simulink model "nouveaux_graphes2"  (R2018a)
settings: Solver=VariableStepAuto  StartTime=0.0  StopTime=100  RelTol=1e-3
settings Model: Creator=acer  LastModifiedBy=ITEC

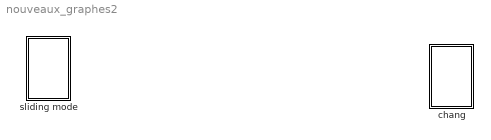
== system nouveaux_graphes2 ==
  chang : Subsystem
  sliding mode : Subsystem

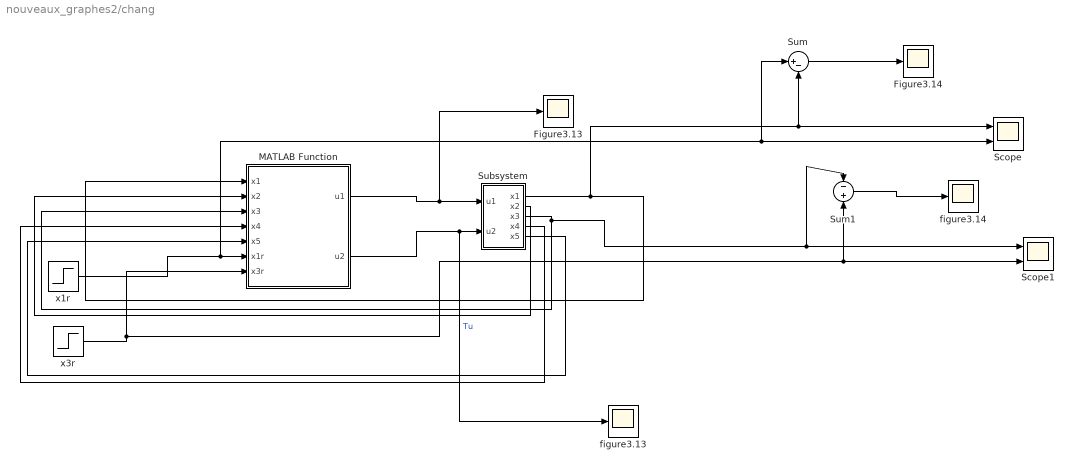
== system nouveaux_graphes2/chang ==
  Figure3.13 : Scope
  Figure3.14 : Scope
  MATLAB Function : MATLAB Function  TreatAsAtomicUnit=on
  Scope : Scope  NumInputPorts=2
  Scope1 : Scope  NumInputPorts=2
  Subsystem : Subsystem
  Sum : Sum  Inputs=|+-
  Sum1 : Sum  Inputs=-+
  figure3.13 : Scope
  figure3.14 : Scope
  x1r : Step  Time=0  After=8*10^6  SampleTime=0
  x3r : Step  Time=0  After=0.36  SampleTime=0
  wires:
  Subsystem/1(x1) -> Sum/2, Scope/1, MATLAB Function/1(x1)
  Subsystem/4(x4) -> MATLAB Function/4(x4)
  Subsystem/5(x5) -> MATLAB Function/5(x5)
  Subsystem/2(x2) -> MATLAB Function/2(x2)
  x1r/1 -> Sum/1, Scope/2, MATLAB Function/6(x1r)
  Sum/1 -> Figure3.14/1
  Subsystem/3(x3) -> Sum1/1, Scope1/1, MATLAB Function/3(x3)
  x3r/1 -> Sum1/2, Scope1/2, MATLAB Function/7(x3r)
  Sum1/1 -> figure3.14/1
  MATLAB Function/1(u1) -> Figure3.13/1, Subsystem/1(u1)
  MATLAB Function/2(u2) -> figure3.13/1, Subsystem/2(u2)  "Tu"

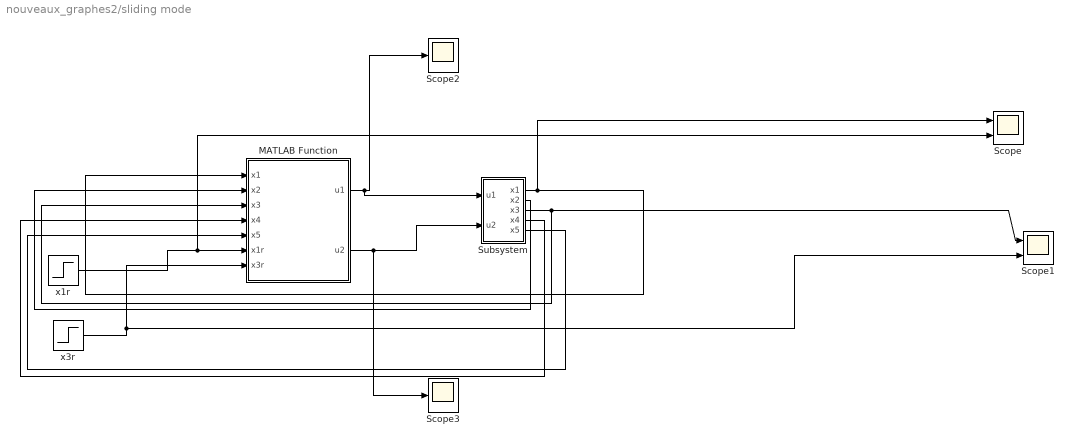
== system nouveaux_graphes2/sliding mode ==
  MATLAB Function : MATLAB Function  TreatAsAtomicUnit=on
  Scope : Scope  NumInputPorts=2
  Scope1 : Scope  NumInputPorts=2
  Scope2 : Scope
  Scope3 : Scope
  Subsystem : Subsystem
  x1r : Step  Time=0  After=8*10^6  SampleTime=0
  x3r : Step  Time=0  After=0.36  SampleTime=0
  wires:
  Subsystem/2(x2) -> MATLAB Function/2(x2)
  Subsystem/1(x1) -> MATLAB Function/1(x1), Scope/1
  MATLAB Function/2(u2) -> Scope3/1, Subsystem/2(u2)
  Subsystem/5(x5) -> MATLAB Function/5(x5)
  x3r/1 -> Scope1/2, MATLAB Function/7(x3r)
  Subsystem/3(x3) -> MATLAB Function/3(x3), Scope1/1
  Subsystem/4(x4) -> MATLAB Function/4(x4)
  x1r/1 -> Scope/2, MATLAB Function/6(x1r)
  MATLAB Function/1(u1) -> Subsystem/1(u1), Scope2/1

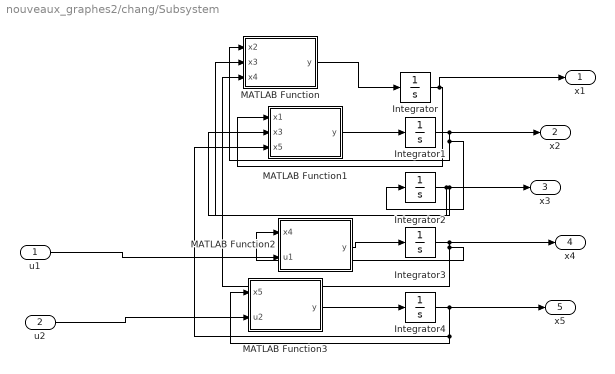
== system nouveaux_graphes2/chang/Subsystem ==
  u1 : Inport
  u2 : Inport  Port=2
  Integrator{,1..4} (5 alike) : Integrator
  MATLAB Function : MATLAB Function  TreatAsAtomicUnit=on
  MATLAB Function1 : MATLAB Function  TreatAsAtomicUnit=on
  MATLAB Function2 : MATLAB Function  TreatAsAtomicUnit=on
  MATLAB Function3 : MATLAB Function  TreatAsAtomicUnit=on
  x1 : Outport
  x2 : Outport  Port=2
  x3 : Outport  Port=3
  x4 : Outport  Port=4
  x5 : Outport  Port=5
  wires:
  Integrator/1 -> x1/1, MATLAB Function1/1(x1)
  Integrator1/1 -> x2/1, Integrator2/1, MATLAB Function/1(x2)
  MATLAB Function3/1(y) -> Integrator4/1
  MATLAB Function1/1(y) -> Integrator1/1
  u1/1 -> MATLAB Function2/2(u1)
  Integrator2/1 -> MATLAB Function1/2(x3), x3/1, MATLAB Function/2(x3)
  Integrator3/1 -> x4/1, MATLAB Function2/1(x4), MATLAB Function/3(x4)
  MATLAB Function2/1(y) -> Integrator3/1
  Integrator4/1 -> x5/1, MATLAB Function3/1(x5), MATLAB Function1/3(x5)
  MATLAB Function/1(y) -> Integrator/1
  u2/1 -> MATLAB Function3/2(u2)

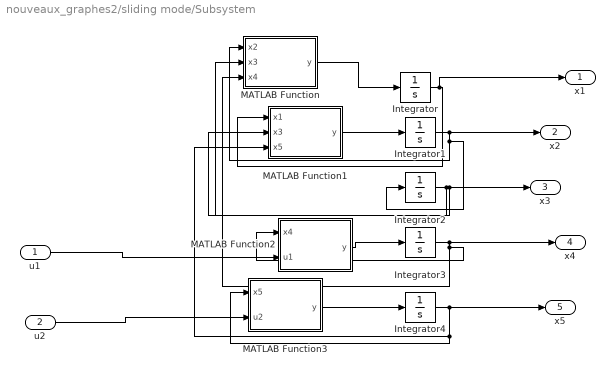
== system nouveaux_graphes2/sliding mode/Subsystem ==
  u1 : Inport
  u2 : Inport  Port=2
  Integrator{,1..4} (5 alike) : Integrator
  MATLAB Function : MATLAB Function  TreatAsAtomicUnit=on
  MATLAB Function1 : MATLAB Function  TreatAsAtomicUnit=on
  MATLAB Function2 : MATLAB Function  TreatAsAtomicUnit=on
  MATLAB Function3 : MATLAB Function  TreatAsAtomicUnit=on
  x1 : Outport
  x2 : Outport  Port=2
  x3 : Outport  Port=3
  x4 : Outport  Port=4
  x5 : Outport  Port=5
  wires:
  Integrator/1 -> x1/1, MATLAB Function1/1(x1)
  Integrator1/1 -> x2/1, Integrator2/1, MATLAB Function/1(x2)
  MATLAB Function3/1(y) -> Integrator4/1
  MATLAB Function1/1(y) -> Integrator1/1
  u1/1 -> MATLAB Function2/2(u1)
  Integrator2/1 -> MATLAB Function1/2(x3), x3/1, MATLAB Function/2(x3)
  Integrator3/1 -> x4/1, MATLAB Function2/1(x4), MATLAB Function/3(x4)
  MATLAB Function2/1(y) -> Integrator3/1
  Integrator4/1 -> x5/1, MATLAB Function3/1(x5), MATLAB Function1/3(x5)
  MATLAB Function/1(y) -> Integrator/1
  u2/1 -> MATLAB Function3/2(u2)

== matlab function nouveaux_graphes2/sliding mode/Subsystem/MATLAB Function1 ==
  data: x1 input; y output; x3 input; x5 input
function y = fcn(x1,x3,x5)
g = 9.8;
rau = 7800;
L = 5.8;
Ml = 1862.9;
RG = 0.194;
J = 172.65;
Rl = 0.611;
H1 = 0.195;
L1 = 2.34;
L4 = 3.46;
Rr=0.0925;
h = 0.00728;
w = 1.5;
A = h*w;
alpha = atan((Rl*sin(x3) - H1 + Rr)/(L1 + Rl*cos(x3)));
beta = atan((Rl*sin(x3) - H1 + Rr)/(L4 - Rl*cos(x3)));
F3 = Rl*(sin(x3+beta) - sin(x3-alpha));
F1 = 0.5*g*rau*L*h*w*Rl*cos(x3) + g*Ml*RG*cos(x3);
y = (x5 - F1 - x1*A*F3)/J;

== matlab function nouveaux_graphes2/sliding mode/Subsystem/MATLAB Function ==
  data: x2 input; y output; x3 input; x4 input
function y = fcn(x2,x3,x4)
E = 1.2*10^10;
L = 5.8;
Rl = 0.611;
H1 = 0.195;
L1 = 2.34;
L4 = 3.46;
Rr=0.0925;
alpha = atan((Rl*sin(x3) - H1 + Rr)/(L1 + Rl*cos(x3)));
beta = atan((Rl*sin(x3) - H1 + Rr)/(L4 - Rl*cos(x3)));
F3 = Rl*(sin(x3+beta) - sin(x3-alpha));
y = E*(F3*x2 - x4)/L;

== matlab function nouveaux_graphes2/sliding mode/Subsystem/MATLAB Function2 ==
  data: x4 input; y output; u1 input
function y = fcn(x4,u1)
TASR = 0.04;
y = (-x4 + u1)/TASR;

== matlab function nouveaux_graphes2/sliding mode/Subsystem/MATLAB Function3 ==
  data: x5 input; y output; u2 input
function y = fcn(x5,u2)
TATR = 0.01;
y = (-x5 + u2)/TATR;

== matlab function nouveaux_graphes2/sliding mode/MATLAB Function ==
  data: x1 input; u1 output; x2 input; x3 input; x4 input; x5 input; x1r input; x3r input; u2 output
function [u1,u2] = fcn(x1,x2,x3,x4,x5,x1r,x3r)
E = 1.2*10^10;
TATR = 0.01;
TASR = 0.04;
g = 9.8;
rau = 7800;
L = 5.8;
Ml = 1862.9;
RG = 0.194;
J = 172.65;
Rl = 0.611;
H1 = 0.195;
L1 = 2.34;
L4 = 3.46;
Rr=0.0925;
h = 0.00728;
w = 1.5;
A = h*w;
lambda1 = 100;% lambda1 = 0.1;
lambda2 = 1;
K = 1;% K = 0.2;
alpha = atan((Rl*sin(x3) - H1 + Rr)/(L1 + Rl*cos(x3)));
beta = atan((Rl*sin(x3) - H1 + Rr)/(L4 - Rl*cos(x3)));
F3 = Rl*(sin(x3+beta) - sin(x3-alpha));
F1 = 0.5*g*rau*L*h*w*Rl*cos(x3) + g*Ml*RG*cos(x3);
F = [E*(F3*x2 - x4)/L;(x5 - F1 - x1*A*F3)/J;x2;-x4/TASR;-x5/TATR];
G = [0 0; 0 0; 0 0; 1/TASR 0; 0 1/TATR];
e1 = x1-x1r;
e2 = x3-x3r;
S1 = lambda1*e1 + F(1);
S2 = lambda2^2*e2 + F(2) + 2*lambda2*x2;
S = [S1;S2];
dF1 = -0.5*g*rau*L*h*w*Rl*sin(x3) -g*Ml*RG*sin(x3);
dF3 = (611*cos(x3 - atan(((611*sin(x3))/1000 - 41/400)/((611*cos(x3))/1000 + 117/50)))*(((611*cos(x3))/(1000*((611*cos(x3))/1000 + 117/50)) + (611*sin(x3)*((611*sin(x3))/1000 - 41/400))/(1000*((611*cos(x3))/1000 + 117/50)^2))/(((611*sin(x3))/1000 - 41/400)^2/((611*cos(x3))/1000 + 117/50)^2 + 1) - 1))/1000 - (611*cos(x3 - atan(((611*sin(x3))/1000 - 41/400)/((611*cos(x3))/1000 - 173/50)))*(((611*cos(x3))/(1000*((611*cos(x3))/1000 - 173/50)) + (611*sin(x3)*((611*sin(x3))/1000 - 41/400))/(1000*((611*cos(x3))/1000 - 173/50)^2))/(((611*sin(x3))/1000 - 41/400)^2/((611*cos(x3))/1000 - 173/50)^2 + 1) - 1))/1000;
dS1 = [lambda1 E*F3/L E*x2*dF3/L -E/L 0];
dS2 = [-A*F3/L 2*lambda2 (lambda2^2)-(dF1 + x1*A*dF3)/J 0 1/J];
dS = [dS1;dS2];
U = inv(dS*G)*(-dS*F -K*sign(S));
u1 = U(1);
u2 = U(2);

== matlab function nouveaux_graphes2/chang/MATLAB Function ==
  data: x1 input; u1 output; x2 input; x3 input; x4 input; x5 input; x1r input; x3r input; u2 output
function [u1,u2] = fcn(x1,x2,x3,x4,x5,x1r,x3r)
E = 1.2*10^10;
TATR = 0.01;
TASR = 0.04;
g = 9.8;
rau = 7800;
L = 5.8;
Ml = 1862.9;
RG = 0.194;
J = 172.65;
Rl = 0.611;
H1 = 0.195;
L1 = 2.34;
L4 = 3.46;
Rr=0.0925;
h = 0.00728;
w = 1.5;
A = h*w;
alpha = atan((Rl*sin(x3) - H1 + Rr)/(L1 + Rl*cos(x3)));
beta = atan((Rl*sin(x3) - H1 + Rr)/(L4 - Rl*cos(x3)));
F3 = Rl*(sin(x3+beta) - sin(x3-alpha));
F1 = 0.5*g*rau*L*h*w*Rl*cos(x3) + g*Ml*RG*cos(x3);
F = [E*(F3*x2 - x4)/L;(x5 - F1 - x1*A*F3)/J;x2;-x4/TASR;-x5/TATR];
G = [0 0; 0 0; 0 0; 1/TASR 0; 0 1/TATR];
dF1 = -0.5*g*rau*L*h*w*Rl*sin(x3) -g*Ml*RG*sin(x3);
dF3 = (611*cos(x3 - atan(((611*sin(x3))/1000 - 41/400)/((611*cos(x3))/1000 + 117/50)))*(((611*cos(x3))/(1000*((611*cos(x3))/1000 + 117/50)) + (611*sin(x3)*((611*sin(x3))/1000 - 41/400))/(1000*((611*cos(x3))/1000 + 117/50)^2))/(((611*sin(x3))/1000 - 41/400)^2/((611*cos(x3))/1000 + 117/50)^2 + 1) - 1))/1000 - (611*cos(x3 - atan(((611*sin(x3))/1000 - 41/400)/((611*cos(x3))/1000 - 173/50)))*(((611*cos(x3))/(1000*((611*cos(x3))/1000 - 173/50)) + (611*sin(x3)*((611*sin(x3))/1000 - 41/400))/(1000*((611*cos(x3))/1000 - 173/50)^2))/(((611*sin(x3))/1000 - 41/400)^2/((611*cos(x3))/1000 - 173/50)^2 + 1) - 1))/1000;
Ax = [-E/(L*TASR) 0; 0 1/(J*TATR)];
A1 = [0 1 0 0 0;0 0 0 0 0;0 0 0 1 0;0 0 0 0 1; 0 0 0 0 0];
B1 = [0 0;1 0;0 0;0 0;0 1];
k = [-1 -2 0 0 0;0 0 -3 -4 -5];
e = [x1-x1r;F(1);x3-x3r;x2;F(2)];
U = inv(Ax)*(-[(E*F3*F(2)/L)+(E*dF3*x2^2/L)+x4*E/(L*TASR);A*F3*F(1)/J-(dF1+x1*A*dF3)*x2/J-x5/(J*TATR)] + k*e);
u1 = U(1);
u2 = U(2);

== matlab function nouveaux_graphes2/chang/Subsystem/MATLAB Function ==
  data: x2 input; y output; x3 input; x4 input
function y = fcn(x2,x3,x4)
E = 1.2*10^10;
L = 5.8;
Rl = 0.611;
H1 = 0.195;
L1 = 2.34;
L4 = 3.46;
Rr=0.0925;
alpha = atan((Rl*sin(x3) - H1 + Rr)/(L1 + Rl*cos(x3)));
beta = atan((Rl*sin(x3) - H1 + Rr)/(L4 - Rl*cos(x3)));
F3 = Rl*(sin(x3+beta) - sin(x3-alpha));
y = E*(F3*x2 - x4)/L;

== matlab function nouveaux_graphes2/chang/Subsystem/MATLAB Function1 ==
  data: x1 input; y output; x3 input; x5 input
function y = fcn(x1,x3,x5)
g = 9.8;
rau = 7800;
L = 5.8;
Ml = 1862.9;
RG = 0.194;
J = 172.65;
Rl = 0.611;
H1 = 0.195;
L1 = 2.34;
L4 = 3.46;
Rr=0.0925;
h = 0.00728;
w = 1.5;
A = h*w;
alpha = atan((Rl*sin(x3) - H1 + Rr)/(L1 + Rl*cos(x3)));
beta = atan((Rl*sin(x3) - H1 + Rr)/(L4 - Rl*cos(x3)));
F3 = Rl*(sin(x3+beta) - sin(x3-alpha));
F1 = 0.5*g*rau*L*h*w*Rl*cos(x3) + g*Ml*RG*cos(x3);
y = (x5 - F1 - x1*A*F3)/J;

== matlab function nouveaux_graphes2/chang/Subsystem/MATLAB Function2 ==
  data: x4 input; y output; u1 input
function y = fcn(x4,u1)
TASR = 0.04;
y = (-x4 + u1)/TASR;

== matlab function nouveaux_graphes2/chang/Subsystem/MATLAB Function3 ==
  data: x5 input; y output; u2 input
function y = fcn(x5,u2)
TATR = 0.01;
y = (-x5 + u2)/TATR;
